simulink model "MPC"  (R2021a)
settings: Solver=ode1  StartTime=0.0  StopTime=10  FixedStep=0.01  RelTol=1e-3
undefined symbols (not defined in the file): DiscIntNeverNeededParam, Kd_psi, Kd_Vx, Ki_psi, Ki_Vx, Kp_psi, Kp_Vx, N, ox, oy, X_0, X_goal, Y_0, Y_goal
libraries: pid_lib x2, simulink x2, slident x2
settings Model: Creator=PC  LastModifiedBy=iris
settings SolverCC: AlgebraicLoopSolver=TrustRegion
settings DebuggingCC: SFMachineParentedDataDiag=warning
settings SFSimCC: CustomCodeUndefinedFunction=UseInterfaceOnly

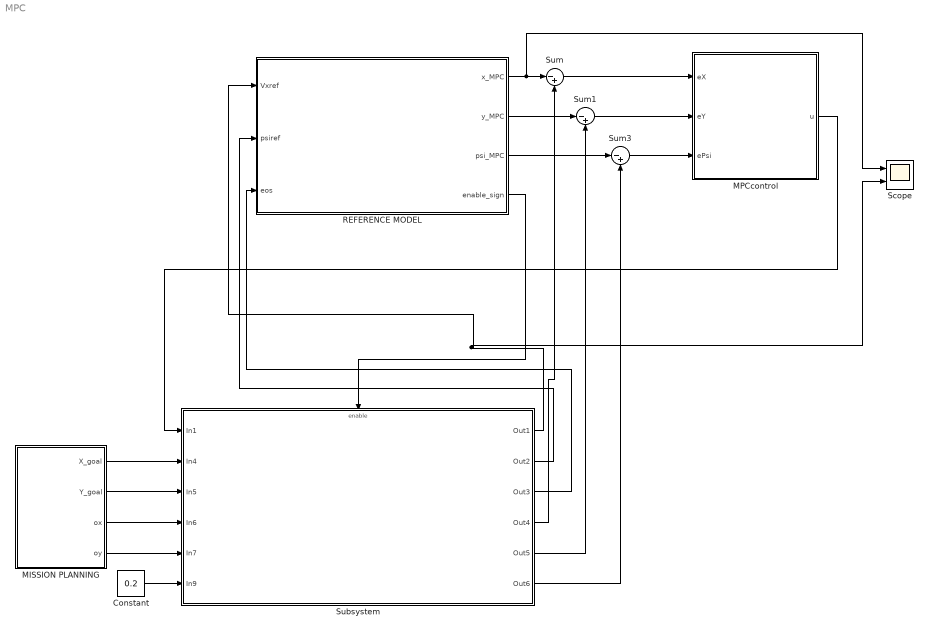
== system MPC ==
  Constant : Constant  Value=0.2
  MISSION PLANNING : Subsystem
  MPCcontrol : Subsystem
  REFERENCE MODEL : Subsystem
  Scope : Scope  NumInputPorts=2
  Subsystem : Subsystem
  Sum : Sum  Inputs=|-+
  Sum1 : Sum  Inputs=|-+
  Sum3 : Sum  Inputs=|-+
  wires:
  REFERENCE MODEL/1(x_MPC) -> Scope/1, Sum/1
  REFERENCE MODEL/2(y_MPC) -> Sum1/1
  REFERENCE MODEL/3(psi_MPC) -> Sum3/1
  Sum/1 -> MPCcontrol/1(eX)
  Sum1/1 -> MPCcontrol/2(eY)
  Sum3/1 -> MPCcontrol/3(ePsi)
  Subsystem/5(Out5) -> Sum1/2
  Subsystem/4(Out4) -> Sum/2
  Subsystem/6(Out6) -> Sum3/2
  MPCcontrol/1(u) -> Subsystem/1(In1)
  MISSION PLANNING/2(Y_goal) -> Subsystem/3(In5)
  MISSION PLANNING/3(ox) -> Subsystem/4(In6)
  MISSION PLANNING/4(oy) -> Subsystem/5(In7)
  Constant/1 -> Subsystem/6(In9)
  Subsystem/1(Out1) -> Scope/2, REFERENCE MODEL/1(Vxref)
  Subsystem/2(Out2) -> REFERENCE MODEL/2(psiref)
  Subsystem/3(Out3) -> REFERENCE MODEL/3(eos)
  REFERENCE MODEL/4(enable_sign) -> Subsystem/Enable
  MISSION PLANNING/1(X_goal) -> Subsystem/2(In4)

== system MPC/MISSION PLANNING ==
  Constant1 : Constant  Value=X_goal
  Constant2 : Constant  Value=Y_goal
  Constant3 : Constant  Value=ox
  Constant4 : Constant  Value=oy
  X_goal : Outport
  Y_goal : Outport  Port=2
  ox : Outport  Port=3
  oy : Outport  Port=4
  wires:
  Constant4/1 -> oy/1
  Constant3/1 -> ox/1
  Constant2/1 -> Y_goal/1
  Constant1/1 -> X_goal/1

== system MPC/MPCcontrol ==
  eX : Inport
  eY : Inport  Port=2
  ePsi : Inport  Port=3
  u : Outport  VectorParamsAs1DForOutWhenUnconnected=off

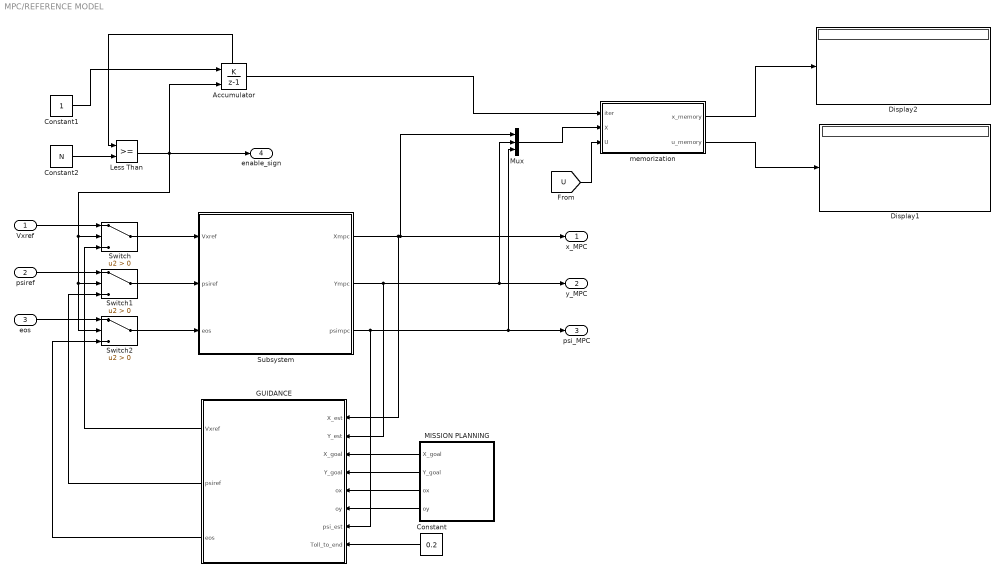
== system MPC/REFERENCE MODEL ==
  Vxref : Inport
  psiref : Inport  Port=2
  eos : Inport  Port=3
  Accumulator : DiscreteIntegrator  IntegratorMethod=Accumulation: Forward Euler  ExternalReset=rising  SampleTime=-1  ShowStatePort=on  ICPrevOutput=DiscIntNeverNeededParam  ICPrevScaledInput=DiscIntNeverNeededParam
  Constant : Constant  Value=0.2
  Constant1 : Constant
  Constant2 : Constant  Value=N
  Display1 : Display
  Display2 : Display
  "GUIDANCE " : Subsystem
  Less Than : RelationalOperator  OutDataTypeStr=boolean  RndMeth=Simplest
  MISSION PLANNING : Subsystem
  Mux : Mux  Inputs=3
  Subsystem : Subsystem
  Switch : Switch  Criteria=u2 > Threshold
  Switch1 : Switch  Criteria=u2 > Threshold
  Switch2 : Switch  Criteria=u2 > Threshold
  memorization : MATLAB Function  TreatAsAtomicUnit=on
  x_MPC : Outport  VectorParamsAs1DForOutWhenUnconnected=off
  y_MPC : Outport  Port=2  VectorParamsAs1DForOutWhenUnconnected=off
  psi_MPC : Outport  Port=3  VectorParamsAs1DForOutWhenUnconnected=off
  enable_sign : Outport  Port=4  VectorParamsAs1DForOutWhenUnconnected=off
  wires:
  Vxref/1 -> Switch/1
  psiref/1 -> Switch1/1
  eos/1 -> Switch2/1
  Switch/1 -> Subsystem/1(Vxref)
  Switch1/1 -> Subsystem/2(psiref)
  "GUIDANCE "/1(Vxref) -> Switch/3
  "GUIDANCE "/2(psiref) -> Switch1/3
  "GUIDANCE "/3(eos) -> Switch2/3
  Switch2/1 -> Subsystem/3(eos)
  Subsystem/2(Ympc) -> Mux/2, y_MPC/1, "GUIDANCE "/2(Y_est)
  MISSION PLANNING/1(X_goal) -> "GUIDANCE "/3(X_goal)
  MISSION PLANNING/2(Y_goal) -> "GUIDANCE "/4(Y_goal)
  MISSION PLANNING/3(ox) -> "GUIDANCE "/5(ox)
  MISSION PLANNING/4(oy) -> "GUIDANCE "/6(oy)
  Constant/1 -> "GUIDANCE "/8(Toll_to_end)
  Accumulator/State -> Less Than/1
  Constant2/1 -> Less Than/2
  Constant1/1 -> Accumulator/1
  Less Than/1 -> Switch/2, Switch1/2, Switch2/2, enable_sign/1, Accumulator/2
  Subsystem/3(psimpc) -> Mux/3, psi_MPC/1, "GUIDANCE "/7(psi_est)
  Subsystem/1(Xmpc) -> "GUIDANCE "/1(X_est), Mux/1, x_MPC/1
  Mux/1 -> memorization/2(X)
  [U] -> memorization/3(U)
  memorization/1(x_memory) -> Display2/1
  memorization/2(u_memory) -> Display1/1
  Accumulator/1 -> memorization/1(iter)

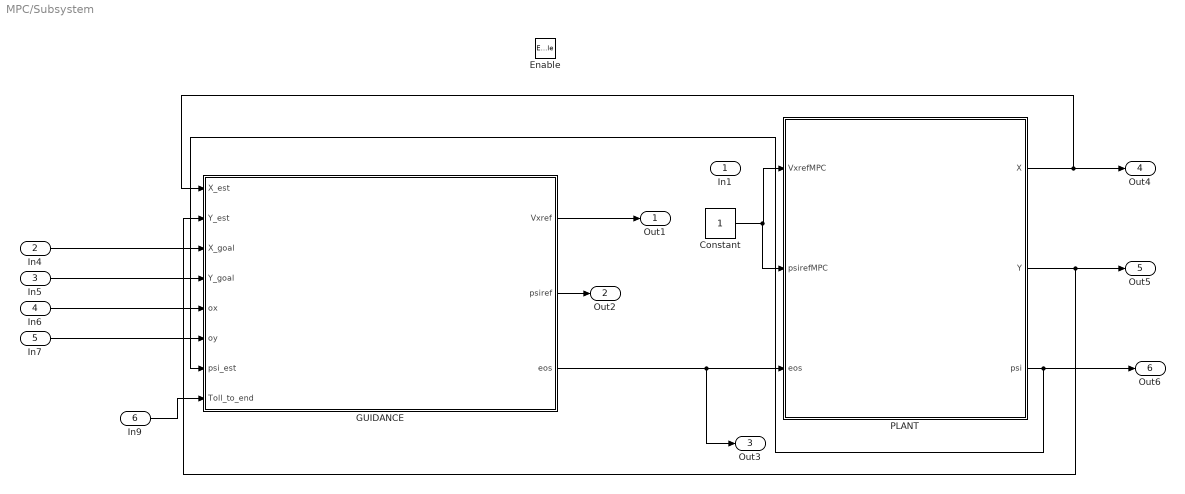
== system MPC/Subsystem ==
  In1 : Inport
  In4 : Inport  Port=2
  In5 : Inport  Port=3
  In6 : Inport  Port=4
  In7 : Inport  Port=5
  In9 : Inport  Port=6
  Enable : EnablePort
  Constant : Constant
  "GUIDANCE " : Subsystem
  PLANT : Subsystem
  Out1 : Outport  VectorParamsAs1DForOutWhenUnconnected=off
  Out2 : Outport  Port=2  VectorParamsAs1DForOutWhenUnconnected=off
  Out3 : Outport  Port=3  VectorParamsAs1DForOutWhenUnconnected=off
  Out4 : Outport  Port=4  VectorParamsAs1DForOutWhenUnconnected=off
  Out5 : Outport  Port=5  VectorParamsAs1DForOutWhenUnconnected=off
  Out6 : Outport  Port=6  VectorParamsAs1DForOutWhenUnconnected=off
  wires:
  PLANT/3(psi) -> "GUIDANCE "/7(psi_est), Out6/1
  PLANT/2(Y) -> "GUIDANCE "/2(Y_est), Out5/1
  PLANT/1(X) -> "GUIDANCE "/1(X_est), Out4/1
  In7/1 -> "GUIDANCE "/6(oy)
  "GUIDANCE "/1(Vxref) -> Out1/1
  In9/1 -> "GUIDANCE "/8(Toll_to_end)
  In4/1 -> "GUIDANCE "/3(X_goal)
  In6/1 -> "GUIDANCE "/5(ox)
  In5/1 -> "GUIDANCE "/4(Y_goal)
  "GUIDANCE "/3(eos) -> Out3/1, PLANT/3(eos)
  "GUIDANCE "/2(psiref) -> Out2/1
  Constant/1 -> PLANT/2(psirefMPC), PLANT/1(VxrefMPC)

== system MPC/REFERENCE MODEL/GUIDANCE  ==
  X_est : Inport
  Y_est : Inport  Port=2
  X_goal : Inport  Port=3
  Y_goal : Inport  Port=4
  ox : Inport  Port=5
  oy : Inport  Port=6
  psi_est : Inport  Port=7
  Toll_to_end : Inport  Port=8
  "GUIDANCE " : Subsystem
  Vxref : Outport
  psiref : Outport  Port=2
  eos : Outport  Port=3  VectorParamsAs1DForOutWhenUnconnected=off
  wires:
  X_est/1 -> "GUIDANCE "/1(X_est)
  X_goal/1 -> "GUIDANCE "/3(X_goal)
  oy/1 -> "GUIDANCE "/6(oy)
  ox/1 -> "GUIDANCE "/5(ox)
  Y_goal/1 -> "GUIDANCE "/4(Y_goal)
  Y_est/1 -> "GUIDANCE "/2(Y_est)
  psi_est/1 -> "GUIDANCE "/7(psi_est)
  Toll_to_end/1 -> "GUIDANCE "/8(Toll_to_end)
  "GUIDANCE "/3(eos) -> eos/1
  "GUIDANCE "/1(Vx_ref) -> Vxref/1
  "GUIDANCE "/2(psi_ref) -> psiref/1

== system MPC/REFERENCE MODEL/MISSION PLANNING ==
  Constant1 : Constant  Value=X_goal
  Constant2 : Constant  Value=Y_goal
  Constant3 : Constant  Value=ox
  Constant4 : Constant  Value=oy
  X_goal : Outport
  Y_goal : Outport  Port=2
  ox : Outport  Port=3
  oy : Outport  Port=4
  wires:
  Constant4/1 -> oy/1
  Constant3/1 -> ox/1
  Constant2/1 -> Y_goal/1
  Constant1/1 -> X_goal/1

== system MPC/REFERENCE MODEL/Subsystem ==
  Vxref : Inport
  psiref : Inport  Port=2
  eos : Inport  Port=3
  "Controll " : Subsystem
  Mux : Mux  Inputs=2
  REFERENCE MODEL : Subsystem
  Xmpc : Outport  VectorParamsAs1DForOutWhenUnconnected=off
  Ympc : Outport  Port=2  VectorParamsAs1DForOutWhenUnconnected=off
  psimpc : Outport  Port=3  VectorParamsAs1DForOutWhenUnconnected=off
  tag scope: U=global
  wires:
  REFERENCE MODEL/1(X_MPC) -> Xmpc/1
  REFERENCE MODEL/2(Y_MPC) -> Ympc/1
  eos/1 -> REFERENCE MODEL/3(eos)
  "Controll "/2(psicmd) -> REFERENCE MODEL/2(psicmd)
  Vxref/1 -> Mux/1, "Controll "/1(Vx_ref)
  REFERENCE MODEL/3(psi_MPC) -> psimpc/1, "Controll "/3(psi)
  psiref/1 -> Mux/2, "Controll "/2(psi_ref)
  REFERENCE MODEL/4(Vx_MPC) -> "Controll "/4(Vx)
  "Controll "/1(Vxcmd) -> REFERENCE MODEL/1(Vxcmd)
  Mux/1 -> [U]

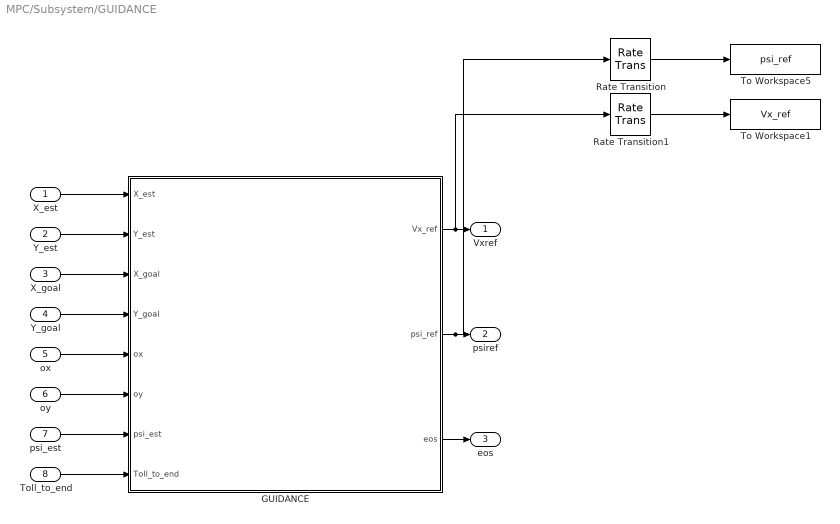
== system MPC/Subsystem/GUIDANCE  ==
  X_est : Inport
  Y_est : Inport  Port=2
  X_goal : Inport  Port=3
  Y_goal : Inport  Port=4
  ox : Inport  Port=5
  oy : Inport  Port=6
  psi_est : Inport  Port=7
  Toll_to_end : Inport  Port=8
  "GUIDANCE " : Subsystem
  Rate Transition : RateTransition
  Rate Transition1 : RateTransition
  To Workspace1 : ToWorkspace  VariableName=Vx_ref  SaveFormat=Structure With Time  SampleTime=-1
  To Workspace5 : ToWorkspace  VariableName=psi_ref  SaveFormat=Structure With Time  SampleTime=-1
  Vxref : Outport
  psiref : Outport  Port=2
  eos : Outport  Port=3  VectorParamsAs1DForOutWhenUnconnected=off
  wires:
  X_est/1 -> "GUIDANCE "/1(X_est)
  X_goal/1 -> "GUIDANCE "/3(X_goal)
  oy/1 -> "GUIDANCE "/6(oy)
  ox/1 -> "GUIDANCE "/5(ox)
  Y_goal/1 -> "GUIDANCE "/4(Y_goal)
  Y_est/1 -> "GUIDANCE "/2(Y_est)
  psi_est/1 -> "GUIDANCE "/7(psi_est)
  Toll_to_end/1 -> "GUIDANCE "/8(Toll_to_end)
  "GUIDANCE "/3(eos) -> eos/1
  Rate Transition/1 -> To Workspace5/1
  "GUIDANCE "/2(psi_ref) -> Rate Transition/1, psiref/1
  "GUIDANCE "/1(Vx_ref) -> Rate Transition1/1, Vxref/1
  Rate Transition1/1 -> To Workspace1/1

== system MPC/Subsystem/PLANT ==
  VxrefMPC : Inport
  psirefMPC : Inport  Port=2
  eos : Inport  Port=3
  PLANT : Subsystem
  X : Outport  VectorParamsAs1DForOutWhenUnconnected=off
  Y : Outport  Port=2  VectorParamsAs1DForOutWhenUnconnected=off
  psi : Outport  Port=3  VectorParamsAs1DForOutWhenUnconnected=off
  wires:
  PLANT/3(psi) -> psi/1
  PLANT/1(X) -> X/1
  VxrefMPC/1 -> PLANT/1(Vxcmd)
  psirefMPC/1 -> PLANT/2(psicmd)
  eos/1 -> PLANT/3(eos)
  PLANT/2(Y) -> Y/1

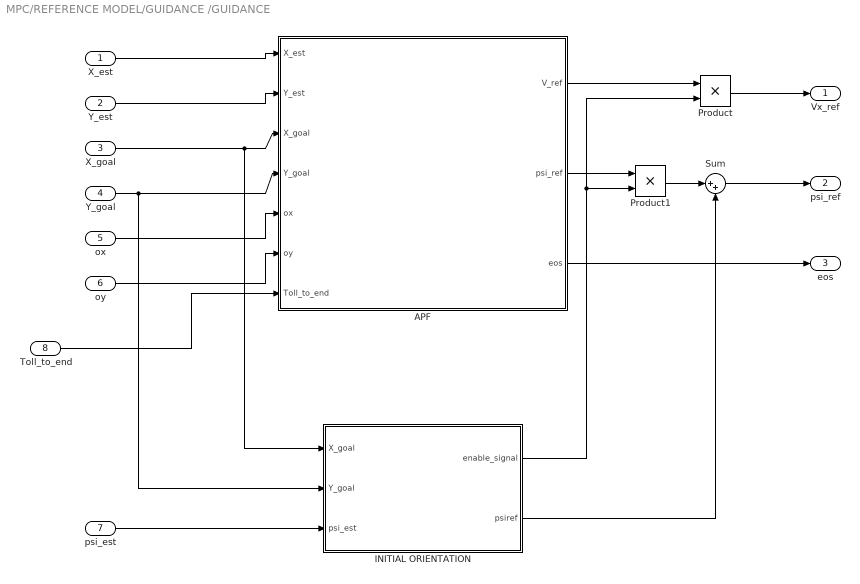
== system MPC/REFERENCE MODEL/GUIDANCE /GUIDANCE  ==
  X_est : Inport
  Y_est : Inport  Port=2
  X_goal : Inport  Port=3
  Y_goal : Inport  Port=4
  ox : Inport  Port=5
  oy : Inport  Port=6
  psi_est : Inport  Port=7
  Toll_to_end : Inport  Port=8
  APF : Subsystem
  INITIAL ORIENTATION : Subsystem
  Product : Product
  Product1 : Product
  Sum : Sum  Inputs=|++
  Vx_ref : Outport
  psi_ref : Outport  Port=2
  eos : Outport  Port=3
  wires:
  X_goal/1 -> INITIAL ORIENTATION/1(X_goal), APF/3(X_goal)
  Y_goal/1 -> INITIAL ORIENTATION/2(Y_goal), APF/4(Y_goal)
  X_est/1 -> APF/1(X_est)
  Y_est/1 -> APF/2(Y_est)
  ox/1 -> APF/5(ox)
  oy/1 -> APF/6(oy)
  Sum/1 -> psi_ref/1
  psi_est/1 -> INITIAL ORIENTATION/3(psi_est)
  INITIAL ORIENTATION/2(psiref) -> Sum/2
  APF/1(V_ref) -> Product/1
  Product/1 -> Vx_ref/1
  INITIAL ORIENTATION/1(enable_signal) -> Product1/2, Product/2
  APF/2(psi_ref) -> Product1/1
  Product1/1 -> Sum/1
  APF/3(eos) -> eos/1
  Toll_to_end/1 -> APF/7(Toll_to_end)

== system MPC/REFERENCE MODEL/Subsystem/Controll  ==
  Vx_ref : Inport
  psi_ref : Inport  Port=2
  psi : Inport  Port=3
  Vx : Inport  Port=4
  Gain : Gain  Gain=180/pi
  Gain2 : Gain  Gain=180/pi
  MATLAB Function : MATLAB Function  TreatAsAtomicUnit=on
  PID Controller : pid_lib/PID Controller  Controller=PID  Form=Parallel  TimeDomain=Discrete-time  UseExternalTs=off  SampleTime=-1  IntegratorMethod=Forward Euler  FilterMethod=Forward Euler  ControllerParametersSource=internal  P=Kp_Vx  I=Ki_Vx  D=Kd_Vx  UseFilter=on  N=100  TunerSelectOption=Transfer Function Based (PID Tuner App)  InitialConditionSource=internal  InitialConditionForIntegrator=0  InitialConditionForFilter=0  DifferentiatorICPrevScaledInput=0  ExternalReset=none  TrackingMode=off  Kt=1  LimitOutput=off  SatLimitsSource=internal  UpperSaturationLimit=inf  LowerSaturationLimit=-inf  LinearizeAsGain=on  AntiWindupMode=none  Kb=1  POutMin=[]  POutMax=[]  IOutMin=[]  IOutMax=[]  DOutMin=[]  DOutMax=[]  NOutMin=[]  NOutMax=[]  SumOutMin=[]  SumOutMax=[]  SaturationOutMin=[]  SaturationOutMax=[]  PParamMin=[]  PParamMax=[]  IParamMin=[]  IParamMax=[]  DParamMin=[]  DParamMax=[]  NParamMin=[]  NParamMax=[]  KbParamMin=[]  KbParamMax=[]  KtParamMin=[]  KtParamMax=[]  KbOutMin=[]  KbOutMax=[]  KtOutMin=[]  KtOutMax=[]  IntegratorOutMin=[]  IntegratorOutMax=[]  FilterOutMin=[]  FilterOutMax=[]  SumI1OutMin=[]  SumI1OutMax=[]  SumI2OutMin=[]  SumI2OutMax=[]  SumI3OutMin=[]  SumI3OutMax=[]  SumI4OutMin=[]  SumI4OutMax=[]  SumDOutMin=[]  SumDOutMax=[]  DifferentiatorOutMin=[]  DifferentiatorOutMax=[]  FilterDiffOutCoefMin=[]  FilterDiffOutCoefMax=[]  ReciprocalOutMin=[]  ReciprocalOutMax=[]  SumDenOutMin=[]  SumDenOutMax=[]  SumNumOutMin=[]  SumNumOutMax=[]  DivideOutMin=[]  DivideOutMax=[]  UdiffTsProdOutMin=[]  UdiffTsProdOutMax=[]  NTsProdOutMin=[]  NTsProdOutMax=[]  UintegralTsProdOutMin=[]  UintegralTsProdOutMax=[]  UngainTsProdOutMin=[]  UngainTsProdOutMax=[]  IntegratorContinuousStateAttributes=''  IntegratorStateMustResolveToSignalObject=off  IntegratorRTWStateStorageClass=Auto  FilterContinuousStateAttributes=''  FilterStateMustResolveToSignalObject=off  FilterRTWStateStorageClass=Auto  ParallelPVariant=InternalParameters  IdealPVariant=Disabled  IVariant=InternalParameters  DVariant=InternalParameters  IntegratorVariant=Discrete  SatVariant=Disabled  AWVariant=Passthrough  PCopyVariant=Disabled  TRVariant=Disabled  FdbkBlocksVariant=Forward  IdealPFdbkVariant=Disabled  SatFdbkVariant=Disabled  DerivativeFilterVariant=ForwardEulerFilter  NVariant=InternalParameters  NCopyVariant=Disabled  FilterICVariant=InternalICsFilter  IntegratorICVariant=InternalICs  ExternalResetVariant=Disabled  TRSumVariant=Passthrough  SumFdbkVariant=Disabled  SumVariant=Sum_PID  TsampFilterVariant=InternalTs  TsampNgainVariant=Passthrough  TsampIntegralVariant=Passthrough  ExternalSaturationOutDataTypeStr=Inherit: Same as second input
  PID Controller1 : pid_lib/PID Controller  Controller=PID  Form=Parallel  TimeDomain=Discrete-time  UseExternalTs=off  SampleTime=-1  IntegratorMethod=Forward Euler  FilterMethod=Forward Euler  ControllerParametersSource=internal  P=Kp_psi  I=Ki_psi  D=Kd_psi  UseFilter=on  N=100  TunerSelectOption=Transfer Function Based (PID Tuner App)  InitialConditionSource=internal  InitialConditionForIntegrator=0  InitialConditionForFilter=0  DifferentiatorICPrevScaledInput=0  ExternalReset=none  TrackingMode=off  Kt=1  LimitOutput=off  SatLimitsSource=internal  UpperSaturationLimit=inf  LowerSaturationLimit=-inf  LinearizeAsGain=on  AntiWindupMode=none  Kb=1  POutMin=[]  POutMax=[]  IOutMin=[]  IOutMax=[]  DOutMin=[]  DOutMax=[]  NOutMin=[]  NOutMax=[]  SumOutMin=[]  SumOutMax=[]  SaturationOutMin=[]  SaturationOutMax=[]  PParamMin=[]  PParamMax=[]  IParamMin=[]  IParamMax=[]  DParamMin=[]  DParamMax=[]  NParamMin=[]  NParamMax=[]  KbParamMin=[]  KbParamMax=[]  KtParamMin=[]  KtParamMax=[]  KbOutMin=[]  KbOutMax=[]  KtOutMin=[]  KtOutMax=[]  IntegratorOutMin=[]  IntegratorOutMax=[]  FilterOutMin=[]  FilterOutMax=[]  SumI1OutMin=[]  SumI1OutMax=[]  SumI2OutMin=[]  SumI2OutMax=[]  SumI3OutMin=[]  SumI3OutMax=[]  SumI4OutMin=[]  SumI4OutMax=[]  SumDOutMin=[]  SumDOutMax=[]  DifferentiatorOutMin=[]  DifferentiatorOutMax=[]  FilterDiffOutCoefMin=[]  FilterDiffOutCoefMax=[]  ReciprocalOutMin=[]  ReciprocalOutMax=[]  SumDenOutMin=[]  SumDenOutMax=[]  SumNumOutMin=[]  SumNumOutMax=[]  DivideOutMin=[]  DivideOutMax=[]  UdiffTsProdOutMin=[]  UdiffTsProdOutMax=[]  NTsProdOutMin=[]  NTsProdOutMax=[]  UintegralTsProdOutMin=[]  UintegralTsProdOutMax=[]  UngainTsProdOutMin=[]  UngainTsProdOutMax=[]  IntegratorContinuousStateAttributes=''  IntegratorStateMustResolveToSignalObject=off  IntegratorRTWStateStorageClass=Auto  FilterContinuousStateAttributes=''  FilterStateMustResolveToSignalObject=off  FilterRTWStateStorageClass=Auto  ParallelPVariant=InternalParameters  IdealPVariant=Disabled  IVariant=InternalParameters  DVariant=InternalParameters  IntegratorVariant=Discrete  SatVariant=Disabled  AWVariant=Passthrough  PCopyVariant=Disabled  TRVariant=Disabled  FdbkBlocksVariant=Forward  IdealPFdbkVariant=Disabled  SatFdbkVariant=Disabled  DerivativeFilterVariant=ForwardEulerFilter  NVariant=InternalParameters  NCopyVariant=Disabled  FilterICVariant=InternalICsFilter  IntegratorICVariant=InternalICs  ExternalResetVariant=Disabled  TRSumVariant=Passthrough  SumFdbkVariant=Disabled  SumVariant=Sum_PID  TsampFilterVariant=InternalTs  TsampNgainVariant=Passthrough  TsampIntegralVariant=Passthrough  ExternalSaturationOutDataTypeStr=Inherit: Same as second input
  Sum : Sum  Inputs=|+-
  Vxcmd : Outport
  psicmd : Outport  Port=2
  wires:
  Gain/1 -> MATLAB Function/1(psi_ref)
  psi_ref/1 -> Gain/1
  Vx_ref/1 -> Sum/1
  Vx/1 -> Sum/2
  psi/1 -> Gain2/1
  Gain2/1 -> MATLAB Function/2(psi_est)
  MATLAB Function/1(errore) -> PID Controller1/1  "psi_error"
  PID Controller1/1 -> psicmd/1
  Sum/1 -> PID Controller/1  "Vx_err"
  PID Controller/1 -> Vxcmd/1

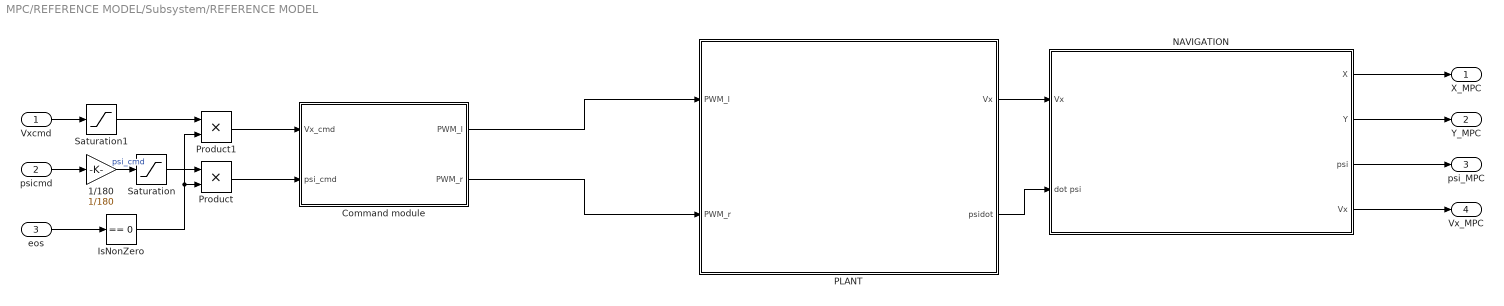
== system MPC/REFERENCE MODEL/Subsystem/REFERENCE MODEL ==
  Vxcmd : Inport
  psicmd : Inport  Port=2
  eos : Inport  Port=3
  1/180 : Gain  Gain=1/180
  Command module : Subsystem
  IsNonZero : simulink/Logic and Bit Operations/Compare To Zero  relop===  OutDataTypeStr=boolean
  NAVIGATION : Subsystem
  PLANT : Subsystem
  Product : Product
  Product1 : Product
  Saturation : Saturate
  Saturation1 : Saturate  UpperLimit=1  LowerLimit=-1
  X_MPC : Outport  VectorParamsAs1DForOutWhenUnconnected=off
  Y_MPC : Outport  Port=2  VectorParamsAs1DForOutWhenUnconnected=off
  psi_MPC : Outport  Port=3  VectorParamsAs1DForOutWhenUnconnected=off
  Vx_MPC : Outport  Port=4  VectorParamsAs1DForOutWhenUnconnected=off
  wires:
  PLANT/2(psidot) -> NAVIGATION/2(dot psi)
  PLANT/1(Vx) -> NAVIGATION/1(Vx)
  Command module/1(PWM_l) -> PLANT/1(PWM_l)
  Command module/2(PWM_r) -> PLANT/2(PWM_r)
  IsNonZero/1 -> Product1/2, Product/2
  1/180/1 -> Saturation/1  "psi_cmd"
  psicmd/1 -> 1/180/1
  Saturation1/1 -> Product1/1
  Saturation/1 -> Product/1
  Vxcmd/1 -> Saturation1/1
  Product1/1 -> Command module/1(Vx_cmd)
  Product/1 -> Command module/2(psi_cmd)
  eos/1 -> IsNonZero/1
  NAVIGATION/4(" Vx") -> Vx_MPC/1
  NAVIGATION/3(psi) -> psi_MPC/1
  NAVIGATION/2(Y) -> Y_MPC/1
  NAVIGATION/1(X) -> X_MPC/1

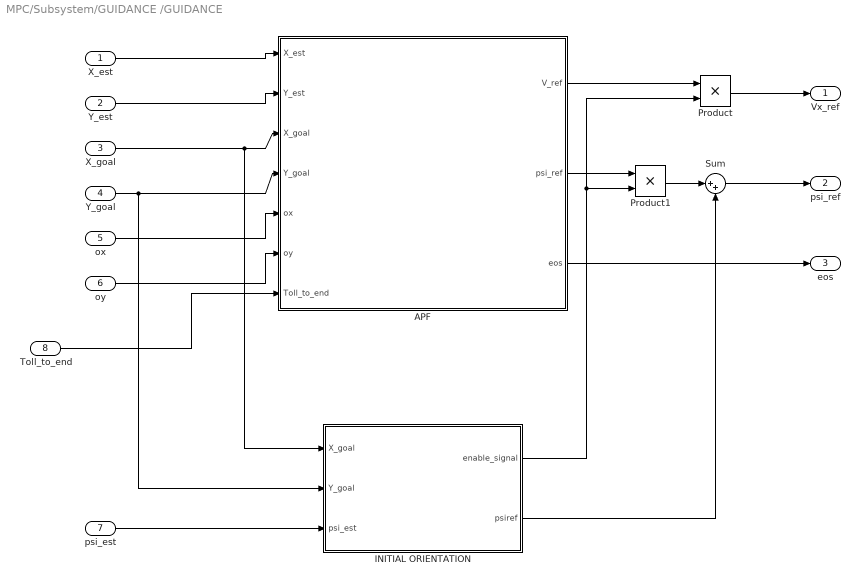
== system MPC/Subsystem/GUIDANCE /GUIDANCE  ==
  X_est : Inport
  Y_est : Inport  Port=2
  X_goal : Inport  Port=3
  Y_goal : Inport  Port=4
  ox : Inport  Port=5
  oy : Inport  Port=6
  psi_est : Inport  Port=7
  Toll_to_end : Inport  Port=8
  APF : Subsystem
  INITIAL ORIENTATION : Subsystem
  Product : Product
  Product1 : Product
  Sum : Sum  Inputs=|++
  Vx_ref : Outport
  psi_ref : Outport  Port=2
  eos : Outport  Port=3
  wires:
  X_goal/1 -> INITIAL ORIENTATION/1(X_goal), APF/3(X_goal)
  Y_goal/1 -> INITIAL ORIENTATION/2(Y_goal), APF/4(Y_goal)
  X_est/1 -> APF/1(X_est)
  Y_est/1 -> APF/2(Y_est)
  ox/1 -> APF/5(ox)
  oy/1 -> APF/6(oy)
  Sum/1 -> psi_ref/1
  psi_est/1 -> INITIAL ORIENTATION/3(psi_est)
  INITIAL ORIENTATION/2(psiref) -> Sum/2
  APF/1(V_ref) -> Product/1
  Product/1 -> Vx_ref/1
  INITIAL ORIENTATION/1(enable_signal) -> Product1/2, Product/2
  APF/2(psi_ref) -> Product1/1
  Product1/1 -> Sum/1
  APF/3(eos) -> eos/1
  Toll_to_end/1 -> APF/7(Toll_to_end)

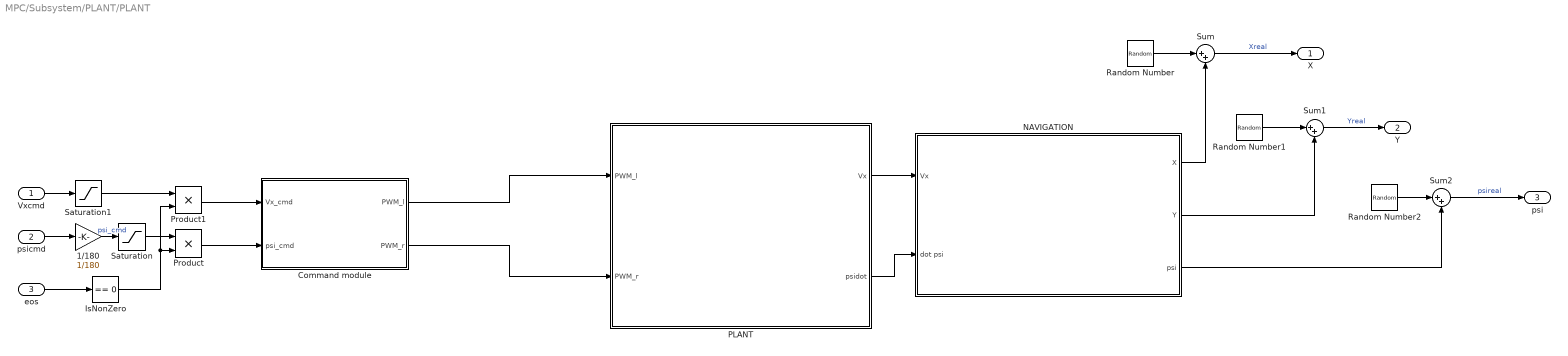
== system MPC/Subsystem/PLANT/PLANT ==
  Vxcmd : Inport
  psicmd : Inport  Port=2
  eos : Inport  Port=3
  1/180 : Gain  Gain=1/180
  Command module : Subsystem
  IsNonZero : simulink/Logic and Bit Operations/Compare To Zero  relop===  OutDataTypeStr=boolean
  NAVIGATION : Subsystem
  PLANT : Subsystem
  Product : Product
  Product1 : Product
  Random Number : RandomNumber  SampleTime=0.1
  Random Number1 : RandomNumber  SampleTime=0.1
  Random Number2 : RandomNumber  SampleTime=0.1
  Saturation : Saturate
  Saturation1 : Saturate  UpperLimit=1  LowerLimit=-1
  Sum : Sum  Inputs=|++
  Sum1 : Sum  Inputs=|++
  Sum2 : Sum  Inputs=|++
  X : Outport  VectorParamsAs1DForOutWhenUnconnected=off
  Y : Outport  Port=2  VectorParamsAs1DForOutWhenUnconnected=off
  psi : Outport  Port=3  VectorParamsAs1DForOutWhenUnconnected=off
  wires:
  PLANT/2(psidot) -> NAVIGATION/2(dot psi)
  PLANT/1(Vx) -> NAVIGATION/1(Vx)
  Random Number/1 -> Sum/1
  Sum/1 -> X/1  "Xreal"
  Sum1/1 -> Y/1  "Yreal"
  Sum2/1 -> psi/1  "psireal"
  Random Number1/1 -> Sum1/1
  Random Number2/1 -> Sum2/1
  NAVIGATION/1(X) -> Sum/2
  NAVIGATION/2(Y) -> Sum1/2
  NAVIGATION/3(psi) -> Sum2/2
  Command module/1(PWM_l) -> PLANT/1(PWM_l)
  Command module/2(PWM_r) -> PLANT/2(PWM_r)
  IsNonZero/1 -> Product1/2, Product/2
  1/180/1 -> Saturation/1  "psi_cmd"
  psicmd/1 -> 1/180/1
  Saturation1/1 -> Product1/1
  Saturation/1 -> Product/1
  Vxcmd/1 -> Saturation1/1
  Product1/1 -> Command module/1(Vx_cmd)
  Product/1 -> Command module/2(psi_cmd)
  eos/1 -> IsNonZero/1

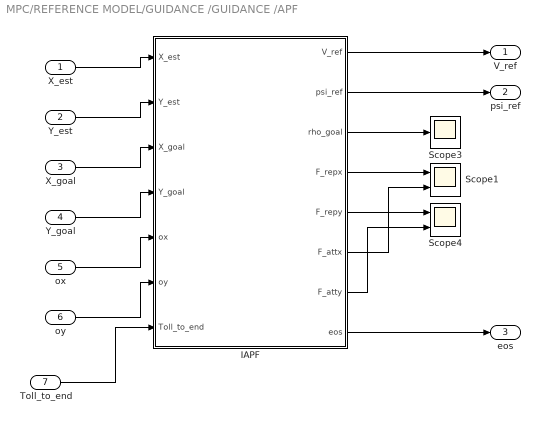
== system MPC/REFERENCE MODEL/GUIDANCE /GUIDANCE /APF ==
  X_est : Inport
  Y_est : Inport  Port=2
  X_goal : Inport  Port=3
  Y_goal : Inport  Port=4
  ox : Inport  Port=5
  oy : Inport  Port=6
  Toll_to_end : Inport  Port=7
  IAPF : MATLAB Function  TreatAsAtomicUnit=on
  Scope1 : Scope  NumInputPorts=2
  Scope3 : Scope
  Scope4 : Scope  NumInputPorts=2
  V_ref : Outport
  psi_ref : Outport  Port=2
  eos : Outport  Port=3
  wires:
  IAPF/1(V_ref) -> V_ref/1
  IAPF/6(F_attx) -> Scope1/2
  IAPF/3(rho_goal) -> Scope3/1
  IAPF/4(F_repx) -> Scope1/1
  IAPF/7(F_atty) -> Scope4/2
  IAPF/5(F_repy) -> Scope4/1
  X_est/1 -> IAPF/1(X_est)
  ox/1 -> IAPF/5(ox)
  IAPF/2(psi_ref) -> psi_ref/1
  Y_est/1 -> IAPF/2(Y_est)
  oy/1 -> IAPF/6(oy)
  IAPF/8(eos) -> eos/1
  X_goal/1 -> IAPF/3(X_goal)
  Y_goal/1 -> IAPF/4(Y_goal)
  Toll_to_end/1 -> IAPF/7(Toll_to_end)

== system MPC/REFERENCE MODEL/GUIDANCE /GUIDANCE /INITIAL ORIENTATION ==
  X_goal : Inport
  Y_goal : Inport  Port=2
  psi_est : Inport  Port=3
  MATLAB Function : MATLAB Function  TreatAsAtomicUnit=on
  enable_signal : Outport
  psiref : Outport  Port=2
  wires:
  psi_est/1 -> MATLAB Function/3(psi_est)
  MATLAB Function/2(psiref) -> psiref/1
  Y_goal/1 -> MATLAB Function/2(Y_goal)
  X_goal/1 -> MATLAB Function/1(X_goal)
  MATLAB Function/1(enable_signal) -> enable_signal/1

== system MPC/REFERENCE MODEL/Subsystem/REFERENCE MODEL/Command module ==
  Vx_cmd : Inport
  psi_cmd : Inport  Port=2
  " " : Gain  Gain=20000
  "   " : Gain  Gain=20000
  Saturation : Saturate  UpperLimit=20000  LowerLimit=-20000
  Saturation1 : Saturate  UpperLimit=20000  LowerLimit=-20000
  Scope : Scope  NumInputPorts=2
  Sum : Sum  Inputs=|++
  Sum1 : Sum  Inputs=|+-
  PWM_l : Outport
  PWM_r : Outport  Port=2
  wires:
  "   "/1 -> Saturation1/1  "pwm_l"
  Sum1/1 -> "   "/1
  Vx_cmd/1 -> Sum/1, Sum1/1
  psi_cmd/1 -> Sum1/2, Sum/2
  Sum/1 -> " "/1
  " "/1 -> Saturation/1  "pwm_r"
  Saturation/1 -> Scope/1, PWM_r/1
  Saturation1/1 -> Scope/2, PWM_l/1

== system MPC/REFERENCE MODEL/Subsystem/REFERENCE MODEL/NAVIGATION ==
  Vx : Inport
  dot psi : Inport  Port=2
  Integrator : Integrator  WrapState=on
  Rate Transition{2..5} (4 alike) : RateTransition  OutPortSampleTime=0.1
  Trasformation block : Subsystem
  X : Outport
  Y : Outport  Port=2
  psi : Outport  Port=3
  " Vx" : Outport  Port=4
  wires:
  dot psi/1 -> Integrator/1
  Rate Transition5/1 -> " Vx"/1
  Trasformation block/1(X) -> Rate Transition3/1
  Trasformation block/2(Y) -> Rate Transition2/1
  Rate Transition4/1 -> psi/1
  Rate Transition2/1 -> Y/1
  Vx/1 -> Rate Transition5/1, Trasformation block/1(Vx)
  Rate Transition3/1 -> X/1
  Integrator/1 -> Rate Transition4/1, Trasformation block/2(psi)

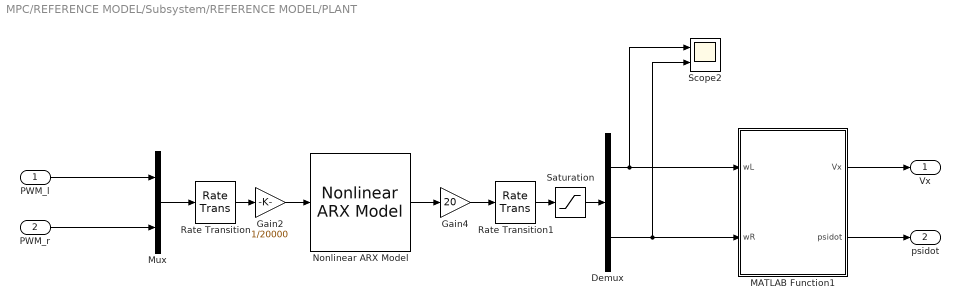
== system MPC/REFERENCE MODEL/Subsystem/REFERENCE MODEL/PLANT ==
  PWM_l : Inport
  PWM_r : Inport  Port=2
  Demux : Demux  Outputs=2
  Gain2 : Gain  Gain=1/20000
  Gain4 : Gain  Gain=20
  MATLAB Function1 : MATLAB Function  TreatAsAtomicUnit=on
  Mux : Mux  Inputs=2
  Nonlinear ARX Model : slident/Models/Nonlinear ARX Model  sys=nlarx1  ICspec=Input and output values  X0=0  U0=0  Y0=0
      settings: SourceProductBaseCode=ID
  Rate Transition : RateTransition
  Rate Transition1 : RateTransition
  Saturation : Saturate  UpperLimit=20  LowerLimit=-20
  Scope2 : Scope  NumInputPorts=2
  Vx : Outport
  psidot : Outport  Port=2
  wires:
  Gain2/1 -> Nonlinear ARX Model/1
  Rate Transition1/1 -> Saturation/1
  Nonlinear ARX Model/1 -> Gain4/1
  MATLAB Function1/1(Vx) -> Vx/1
  Rate Transition/1 -> Gain2/1
  Demux/2 -> Scope2/2, MATLAB Function1/2(wR)
  Mux/1 -> Rate Transition/1
  Demux/1 -> Scope2/1, MATLAB Function1/1(wL)
  Gain4/1 -> Rate Transition1/1
  PWM_r/1 -> Mux/2
  MATLAB Function1/2(psidot) -> psidot/1
  PWM_l/1 -> Mux/1
  Saturation/1 -> Demux/1

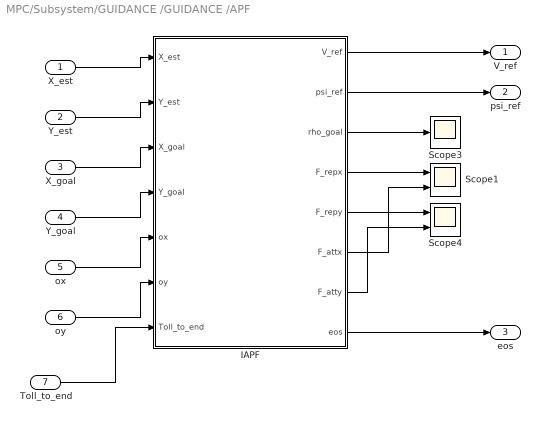
== system MPC/Subsystem/GUIDANCE /GUIDANCE /APF ==
  X_est : Inport
  Y_est : Inport  Port=2
  X_goal : Inport  Port=3
  Y_goal : Inport  Port=4
  ox : Inport  Port=5
  oy : Inport  Port=6
  Toll_to_end : Inport  Port=7
  IAPF : MATLAB Function  TreatAsAtomicUnit=on
  Scope1 : Scope  NumInputPorts=2
  Scope3 : Scope
  Scope4 : Scope  NumInputPorts=2
  V_ref : Outport
  psi_ref : Outport  Port=2
  eos : Outport  Port=3
  wires:
  IAPF/1(V_ref) -> V_ref/1
  IAPF/6(F_attx) -> Scope1/2
  IAPF/3(rho_goal) -> Scope3/1
  IAPF/4(F_repx) -> Scope1/1
  IAPF/7(F_atty) -> Scope4/2
  IAPF/5(F_repy) -> Scope4/1
  X_est/1 -> IAPF/1(X_est)
  ox/1 -> IAPF/5(ox)
  IAPF/2(psi_ref) -> psi_ref/1
  Y_est/1 -> IAPF/2(Y_est)
  oy/1 -> IAPF/6(oy)
  IAPF/8(eos) -> eos/1
  X_goal/1 -> IAPF/3(X_goal)
  Y_goal/1 -> IAPF/4(Y_goal)
  Toll_to_end/1 -> IAPF/7(Toll_to_end)

== system MPC/Subsystem/GUIDANCE /GUIDANCE /INITIAL ORIENTATION ==
  X_goal : Inport
  Y_goal : Inport  Port=2
  psi_est : Inport  Port=3
  MATLAB Function : MATLAB Function  TreatAsAtomicUnit=on
  enable_signal : Outport
  psiref : Outport  Port=2
  wires:
  psi_est/1 -> MATLAB Function/3(psi_est)
  MATLAB Function/2(psiref) -> psiref/1
  Y_goal/1 -> MATLAB Function/2(Y_goal)
  X_goal/1 -> MATLAB Function/1(X_goal)
  MATLAB Function/1(enable_signal) -> enable_signal/1

== system MPC/Subsystem/PLANT/PLANT/Command module ==
  Vx_cmd : Inport
  psi_cmd : Inport  Port=2
  " " : Gain  Gain=20000
  "   " : Gain  Gain=20000
  Saturation : Saturate  UpperLimit=20000  LowerLimit=-20000
  Saturation1 : Saturate  UpperLimit=20000  LowerLimit=-20000
  Scope : Scope  NumInputPorts=2
  Sum : Sum  Inputs=|++
  Sum1 : Sum  Inputs=|+-
  PWM_l : Outport
  PWM_r : Outport  Port=2
  wires:
  "   "/1 -> Saturation1/1  "pwm_l"
  Sum1/1 -> "   "/1
  Vx_cmd/1 -> Sum/1, Sum1/1
  psi_cmd/1 -> Sum1/2, Sum/2
  Sum/1 -> " "/1
  " "/1 -> Saturation/1  "pwm_r"
  Saturation/1 -> Scope/1, PWM_r/1
  Saturation1/1 -> Scope/2, PWM_l/1

== system MPC/Subsystem/PLANT/PLANT/NAVIGATION ==
  Vx : Inport
  dot psi : Inport  Port=2
  Integrator : Integrator  WrapState=on
  Rate Transition2 : RateTransition  OutPortSampleTime=0.1
  Rate Transition3 : RateTransition  OutPortSampleTime=0.1
  Rate Transition4 : RateTransition  OutPortSampleTime=0.1
  Trasformation block : Subsystem
  X : Outport
  Y : Outport  Port=2
  psi : Outport  Port=3
  wires:
  dot psi/1 -> Trasformation block/1(dot psi), Integrator/1
  Trasformation block/1(X) -> Rate Transition3/1
  Trasformation block/2(Y) -> Rate Transition2/1
  Rate Transition4/1 -> psi/1
  Rate Transition2/1 -> Y/1
  Vx/1 -> Trasformation block/2(Vx)
  Rate Transition3/1 -> X/1
  Integrator/1 -> Rate Transition4/1, Trasformation block/3(psi)

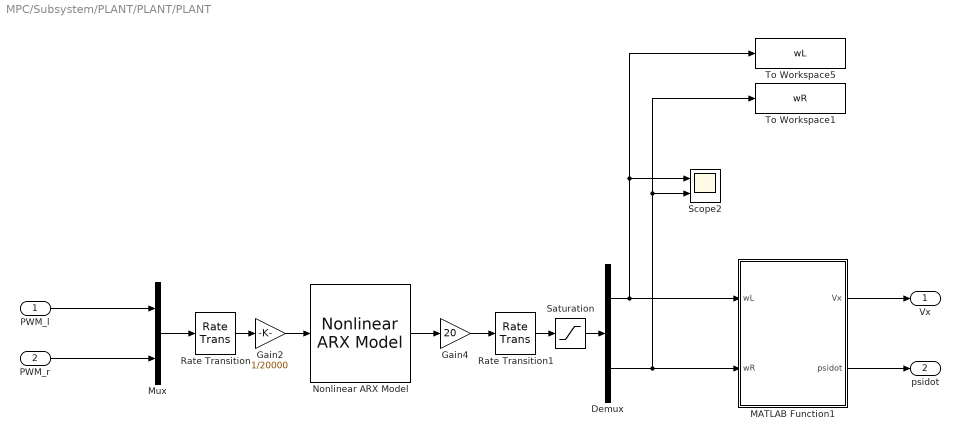
== system MPC/Subsystem/PLANT/PLANT/PLANT ==
  PWM_l : Inport
  PWM_r : Inport  Port=2
  Demux : Demux  Outputs=2
  Gain2 : Gain  Gain=1/20000
  Gain4 : Gain  Gain=20
  MATLAB Function1 : MATLAB Function  TreatAsAtomicUnit=on
  Mux : Mux  Inputs=2
  Nonlinear ARX Model : slident/Models/Nonlinear ARX Model  sys=nlarx1  ICspec=Input and output values  X0=0  U0=0  Y0=0
      settings: SourceProductBaseCode=ID
  Rate Transition : RateTransition
  Rate Transition1 : RateTransition
  Saturation : Saturate  UpperLimit=20  LowerLimit=-20
  Scope2 : Scope  NumInputPorts=2
  To Workspace1 : ToWorkspace  VariableName=wR  SaveFormat=Structure With Time  SampleTime=-1
  To Workspace5 : ToWorkspace  VariableName=wL  SaveFormat=Structure With Time  SampleTime=-1
  Vx : Outport
  psidot : Outport  Port=2
  wires:
  Gain2/1 -> Nonlinear ARX Model/1
  Rate Transition1/1 -> Saturation/1
  Nonlinear ARX Model/1 -> Gain4/1
  MATLAB Function1/1(Vx) -> Vx/1
  Rate Transition/1 -> Gain2/1
  Demux/2 -> Scope2/2, To Workspace1/1, MATLAB Function1/2(wR)
  Mux/1 -> Rate Transition/1
  Demux/1 -> Scope2/1, To Workspace5/1, MATLAB Function1/1(wL)
  Gain4/1 -> Rate Transition1/1
  PWM_r/1 -> Mux/2
  MATLAB Function1/2(psidot) -> psidot/1
  PWM_l/1 -> Mux/1
  Saturation/1 -> Demux/1

== system MPC/REFERENCE MODEL/Subsystem/REFERENCE MODEL/NAVIGATION/Trasformation block ==
  Vx : Inport
  psi : Inport  Port=2
  Integrator5 : Integrator  InitialCondition=X_0
  Integrator7 : Integrator  InitialCondition=Y_0
  MATLAB Function : MATLAB Function  TreatAsAtomicUnit=on
  X : Outport
  Y : Outport  Port=2
  wires:
  psi/1 -> MATLAB Function/2(psi)
  MATLAB Function/1(VX) -> Integrator5/1  "Xdot"
  Vx/1 -> MATLAB Function/1(Vx)
  Integrator7/1 -> Y/1  "Y"
  MATLAB Function/2(VY) -> Integrator7/1  "Ydot"
  Integrator5/1 -> X/1  "X"

== system MPC/Subsystem/PLANT/PLANT/NAVIGATION/Trasformation block ==
  dot psi : Inport
  Vx : Inport  Port=2
  psi : Inport  Port=3
  Integrator5 : Integrator  InitialCondition=X_0
  Integrator7 : Integrator  InitialCondition=Y_0
  MATLAB Function : MATLAB Function  TreatAsAtomicUnit=on
  To Workspace : ToWorkspace  VariableName=X  SaveFormat=Structure With Time  SampleTime=-1
  To Workspace1 : ToWorkspace  VariableName=Y  SaveFormat=Structure With Time  SampleTime=-1
  To Workspace2 : ToWorkspace  VariableName=Xdot  SaveFormat=Structure With Time  SampleTime=-1
  To Workspace3 : ToWorkspace  VariableName=Ydot  SaveFormat=Structure With Time  SampleTime=-1
  To Workspace4 : ToWorkspace  VariableName=psi  SaveFormat=Structure With Time  SampleTime=-1
  To Workspace5 : ToWorkspace  VariableName=psidot  SaveFormat=Structure With Time  SampleTime=-1
  X : Outport
  Y : Outport  Port=2
  wires:
  psi/1 -> To Workspace4/1, MATLAB Function/2(psi)
  MATLAB Function/1(VX) -> To Workspace2/1, Integrator5/1  "Xdot"
  Vx/1 -> MATLAB Function/1(Vx)
  Integrator7/1 -> Y/1, To Workspace1/1  "Y"
  MATLAB Function/2(VY) -> To Workspace3/1, Integrator7/1  "Ydot"
  Integrator5/1 -> X/1, To Workspace/1  "X"
  dot psi/1 -> To Workspace5/1

== matlab function MPC/REFERENCE MODEL/Subsystem/REFERENCE MODEL/PLANT/MATLAB Function1 ==
  data: wL input; Vx output; wR input; psidot output
function [Vx, psidot] = fcn(wL, wR)
r=0.043/2;
B=0.185;

Vx=(wR+wL)*r/2;
psidot=(wR-wL)*r/B;

== matlab function MPC/REFERENCE MODEL/GUIDANCE /GUIDANCE /APF/IAPF ==
  data: X_est input; V_ref output; Y_est input; X_goal input; Y_goal input; ox input; oy input; psi_ref output; rho_goal output; F_repx output; F_repy output; F_attx output; F_atty output; eos output; Toll_to_end input
function [V_ref, psi_ref, rho_goal, F_repx, F_repy, F_attx, F_atty, eos]  = fcn(X_est, Y_est, X_goal, Y_goal,  ox, oy, Toll_to_end)

% Potential field characteristics
rho_0=0.7;                   % Area of influence of obstacle  [m]
kp = 0.15;                   % Attractive pottential gain
eta = 0.05;                  % Repulsive potential gain

q=[X_est, Y_est]';           % Actual position [m]       
qg=[X_goal, Y_goal]';        % Goal position   [m]
rho_goal=norm(q-qg,2);       % Distance actual position-goal position
d=2;                         % Distance from goal, point of attractive field characteristic switching

% ATTRACTIVE
if rho_goal<=d
F_attx = -kp*(X_est-X_goal);
F_atty = -kp*(Y_est-Y_goal);
else    
F_attx = -kp*(X_est-X_goal)*d/rho_goal;
F_atty = -kp*(Y_est-Y_goal)*d/rho_goal;
end


% REPULSIVE
F_repx=0;
F_repy=0;
dmin=10000;
qc=[0 0]';
obst=0;

for k=1:length(ox)
    qc=[ox(k) oy(k)]';                          % Obstacle position [m]
    dq = norm(q-qc,2);                          % Distance actual position- obstacle position
     
    if dmin >= dq
        dmin = dq;
        min_ost = k;
        qc=[ox(min_ost) oy(min_ost)]';
        rho = norm(q-qc,2) ;                    % Distance with the nearest obstacle
        
        if rho<=rho_0                           % Inside obstacle area! Danger
           F_repx=eta*(1/rho - 1/rho_0)*1/(rho).^2*(X_est-ox(min_ost))/norm(q-qc,2);
           F_repy=eta*(1/rho - 1/rho_0)*1/(rho).^2*(Y_est-oy(min_ost))/norm(q-qc,2);  
           obst=1/rho;
        end
     
     end
end

% To find the goal if the obstacle is near
dob=0.3;
dgr=0.3;

if norm(qg-qc,2)<=dob && norm(q-qg,2)<=dgr
    F_totx=F_attx;
    F_toty=F_atty;
else
    F_totx = F_attx+F_repx;
    F_toty = F_atty+F_repy;
end

% Potential Force
F_tot=norm([F_totx,F_toty]);


% ORIENTATION REFERENCE SIGNAL
psi_ref=atan2(F_toty,F_totx);


% VELOCITY REFERENCE SIGNAL
% 1° prova per il campo di velocità
% V_ref=F_totx/F_tot*0.3;

% 2° prova per il campo di velocità
delta=0.4/rho_goal+obst;
V_ref= 0.3*2/(2+delta);

eos = 0;
% END OF SIMULATION
if abs(rho_goal)<=Toll_to_end
    eos=1;
end

% Mathematical minimum
if F_tot==0
    psi_ref=0;
    V_ref=-0.3;
end

== matlab function MPC/REFERENCE MODEL/GUIDANCE /GUIDANCE /INITIAL ORIENTATION/MATLAB Function ==
  data: X_goal input; enable_signal output; Y_goal input; psi_est input; psiref output
function [enable_signal, psiref] = fcn(X_goal, Y_goal, psi_est)
psiref=0;
enable_signal=0;

persistent en
if isempty(en)
    en=0;
end

if en==0
if -pi<psi_est && psi_est<=-pi/2 
  if X_goal>=0 && Y_goal>=0
      enable_signal=0;
      psiref=0;
      en=0;
  end
   if X_goal>0 && Y_goal<0
      enable_signal=0;
      psiref=0;
      en=0;
   end
    if X_goal<=0 && Y_goal<=0
      enable_signal=1;
      en=1;
      psiref=0;
    end
    if X_goal<0 && Y_goal>0
      enable_signal=1;
      en=1;
      psiref=0;
    end
end
if pi/2<psi_est && psi_est<=pi 
  if X_goal>=0 && Y_goal>=0
      enable_signal=0;
      psiref=0;
      en=0;
  end
   if X_goal>0 && Y_goal<0
      enable_signal=0;
      psiref=0;
      en=0;
   end
    if X_goal<=0 && Y_goal<=0
      enable_signal=1;
      en=1;
      psiref=0;
    end
    if X_goal<0 && Y_goal>0
      enable_signal=1;
      en=1;
      psiref=0;
    end
end

if -pi/2<=psi_est && psi_est<=pi/2
  if X_goal>=0 && Y_goal>=0
      enable_signal=1;
      en=1;
      psiref=0;
  end
   if X_goal>0 && Y_goal<0
      enable_signal=1;
      en=1;
      psiref=0;
   end
    if X_goal<=0 && Y_goal<=0
      enable_signal=0;
      psiref=-pi;
      en=0;
    end
    if X_goal<0 && Y_goal>0
      enable_signal=0;
      psiref=pi;
      en=0;
    end
end
else
    enable_signal=1;
    psiref=0;
end

== matlab function MPC/REFERENCE MODEL/memorization ==
  data: iter input; x_memory output; X input; U input; u_memory output
function [x_memory,u_memory] = fcn(iter,X,U)


persistent x_vector;
persistent u_vector;

if isempty(x_vector)
    x_vector = zeros(5,3);
end
if isempty(u_vector)
    u_vector = zeros(5,2);
end

if iter+1 == 6
    x_vector = zeros(5,3);
    u_vector = zeros(5,2);

end

x_vector(iter+1,:) = X;
u_vector(iter+1,:) = U;

x_memory = x_vector;
u_memory = u_vector;

end

== matlab function MPC/Subsystem/GUIDANCE /GUIDANCE /INITIAL ORIENTATION/MATLAB Function ==
  data: X_goal input; enable_signal output; Y_goal input; psi_est input; psiref output
function [enable_signal, psiref] = fcn(X_goal, Y_goal, psi_est)
psiref=0;
enable_signal=0;

persistent en
if isempty(en)
    en=0;
end

if en==0
if -pi<psi_est && psi_est<=-pi/2 
  if X_goal>=0 && Y_goal>=0
      enable_signal=0;
      psiref=0;
      en=0;
  end
   if X_goal>0 && Y_goal<0
      enable_signal=0;
      psiref=0;
      en=0;
   end
    if X_goal<=0 && Y_goal<=0
      enable_signal=1;
      en=1;
      psiref=0;
    end
    if X_goal<0 && Y_goal>0
      enable_signal=1;
      en=1;
      psiref=0;
    end
end
if pi/2<psi_est && psi_est<=pi 
  if X_goal>=0 && Y_goal>=0
      enable_signal=0;
      psiref=0;
      en=0;
  end
   if X_goal>0 && Y_goal<0
      enable_signal=0;
      psiref=0;
      en=0;
   end
    if X_goal<=0 && Y_goal<=0
      enable_signal=1;
      en=1;
      psiref=0;
    end
    if X_goal<0 && Y_goal>0
      enable_signal=1;
      en=1;
      psiref=0;
    end
end

if -pi/2<=psi_est && psi_est<=pi/2
  if X_goal>=0 && Y_goal>=0
      enable_signal=1;
      en=1;
      psiref=0;
  end
   if X_goal>0 && Y_goal<0
      enable_signal=1;
      en=1;
      psiref=0;
   end
    if X_goal<=0 && Y_goal<=0
      enable_signal=0;
      psiref=-pi;
      en=0;
    end
    if X_goal<0 && Y_goal>0
      enable_signal=0;
      psiref=pi;
      en=0;
    end
end
else
    enable_signal=1;
    psiref=0;
end

== matlab function MPC/Subsystem/PLANT/PLANT/PLANT/MATLAB Function1 ==
  data: wL input; Vx output; wR input; psidot output
function [Vx, psidot] = fcn(wL, wR)
r=0.043/2;
B=0.185;

Vx=(wR+wL)*r/2;
psidot=(wR-wL)*r/B;

== matlab function MPC/Subsystem/PLANT/PLANT/NAVIGATION/Trasformation block/MATLAB Function ==
  data: Vx input; VX output; psi input; VY output
function [VX, VY] = fcn(Vx, psi)

M=[cos(psi) -sin(psi); sin(psi) cos(psi)];

X=M*Vx;
VX=X(1);
VY=X(2);

== matlab function MPC/REFERENCE MODEL/Subsystem/REFERENCE MODEL/NAVIGATION/Trasformation block/MATLAB Function ==
  data: Vx input; VX output; psi input; VY output
function [VX, VY] = fcn(Vx, psi)

M=[cos(psi) -sin(psi); sin(psi) cos(psi)];

X=M*Vx;
VX=X(1);
VY=X(2);

== matlab function MPC/REFERENCE MODEL/Subsystem/Controll /MATLAB Function ==
  data: psi_ref input; errore output; psi_est input
function errore = fcn(psi_ref, psi_est)
errore=psi_ref-psi_est;

if abs(errore)>180
    errore=errore-360*sign(errore);
end

== matlab function MPC/Subsystem/GUIDANCE /GUIDANCE /APF/IAPF ==
  data: X_est input; V_ref output; Y_est input; X_goal input; Y_goal input; ox input; oy input; psi_ref output; rho_goal output; F_repx output; F_repy output; F_attx output; F_atty output; eos output; Toll_to_end input
function [V_ref, psi_ref, rho_goal, F_repx, F_repy, F_attx, F_atty, eos]  = fcn(X_est, Y_est, X_goal, Y_goal,  ox, oy, Toll_to_end)

% Potential field characteristics
rho_0=0.7;                   % Area of influence of obstacle  [m]
kp = 0.15;                   % Attractive pottential gain
eta = 0.05;                  % Repulsive potential gain

q=[X_est, Y_est]';           % Actual position [m]       
qg=[X_goal, Y_goal]';        % Goal position   [m]
rho_goal=norm(q-qg,2);       % Distance actual position-goal position
d=2;                         % Distance from goal, point of attractive field characteristic switching

% ATTRACTIVE
if rho_goal<=d
F_attx = -kp*(X_est-X_goal);
F_atty = -kp*(Y_est-Y_goal);
else    
F_attx = -kp*(X_est-X_goal)*d/rho_goal;
F_atty = -kp*(Y_est-Y_goal)*d/rho_goal;
end


% REPULSIVE
F_repx=0;
F_repy=0;
dmin=10000;
qc=[0 0]';
obst=0;

for k=1:length(ox)
    qc=[ox(k) oy(k)]';                          % Obstacle position [m]
    dq = norm(q-qc,2);                          % Distance actual position- obstacle position
     
    if dmin >= dq
        dmin = dq;
        min_ost = k;
        qc=[ox(min_ost) oy(min_ost)]';
        rho = norm(q-qc,2) ;                    % Distance with the nearest obstacle
        
        if rho<=rho_0                           % Inside obstacle area! Danger
           F_repx=eta*(1/rho - 1/rho_0)*1/(rho).^2*(X_est-ox(min_ost))/norm(q-qc,2);
           F_repy=eta*(1/rho - 1/rho_0)*1/(rho).^2*(Y_est-oy(min_ost))/norm(q-qc,2);  
           obst=1/rho;
        end
     
     end
end

% To find the goal if the obstacle is near
dob=0.3;
dgr=0.3;

if norm(qg-qc,2)<=dob && norm(q-qg,2)<=dgr
    F_totx=F_attx;
    F_toty=F_atty;
else
    F_totx = F_attx+F_repx;
    F_toty = F_atty+F_repy;
end

% Potential Force
F_tot=norm([F_totx,F_toty]);


% ORIENTATION REFERENCE SIGNAL
psi_ref=atan2(F_toty,F_totx);


% VELOCITY REFERENCE SIGNAL
% 1° prova per il campo di velocità
% V_ref=F_totx/F_tot*0.3;

% 2° prova per il campo di velocità
delta=0.4/rho_goal+obst;
V_ref= 0.3*2/(2+delta);

eos = 0;
% END OF SIMULATION
if abs(rho_goal)<=Toll_to_end
    eos=1;
end

% Mathematical minimum
if F_tot==0
    psi_ref=0;
    V_ref=-0.3;
end
